simulink model "ProcessFlowRateModel_symbotic"  (Simulink 7.9)
settings: Solver=VariableStepDiscrete  StartTime=0.0  StopTime=100000  RelTol=1e-3
libraries: simeventslib x4
settings Model: Creator=tsprock3  LastModifiedBy=tsprock3
settings DebuggingCC: SimStateOlderReleaseMsg=warning

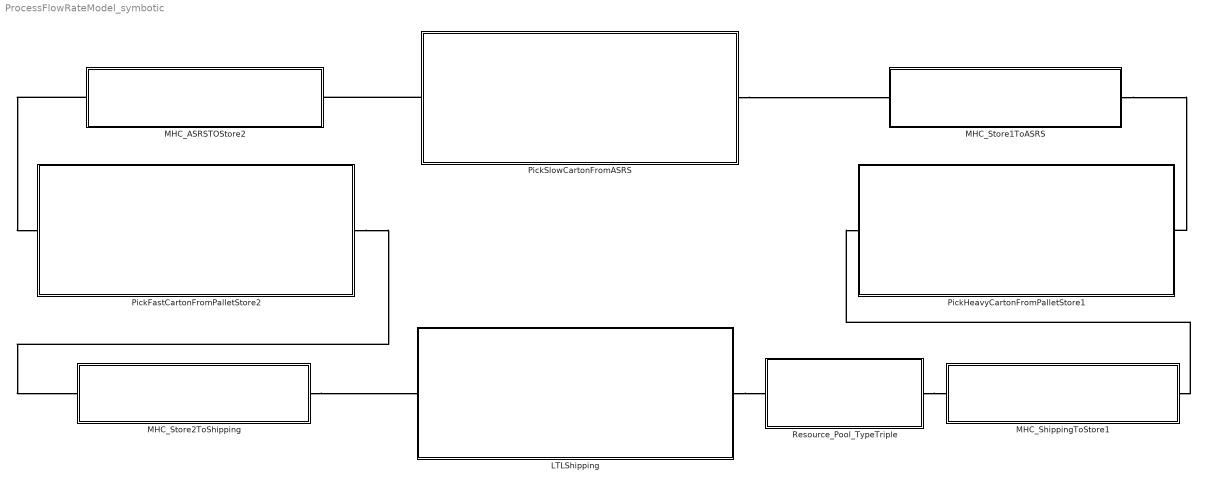
== system ProcessFlowRateModel_symbotic ==
  LTLShipping : Subsystem
  MHC_ASRSTOStore2 : Subsystem
  MHC_ShippingToStore1 : Subsystem
  MHC_Store1ToASRS : Subsystem
  MHC_Store2ToShipping : Subsystem
  PickFastCartonFromPalletStore2 : Subsystem
  PickHeavyCartonFromPalletStore1 : Subsystem
  PickSlowCartonFromASRS : Subsystem
  Resource_Pool_TypeTriple : Subsystem  mask{Quantity=25}
      mask prompts: Quantity "How many entities in resource pool?"
  connections:
  MHC_Store2ToShipping/RConn1 -- LTLShipping/LConn1
  MHC_ShippingToStore1/RConn1 -- PickHeavyCartonFromPalletStore1/LConn1
  MHC_Store1ToASRS/LConn1 -- PickHeavyCartonFromPalletStore1/RConn1
  PickFastCartonFromPalletStore2/RConn1 -- MHC_Store2ToShipping/LConn1
  MHC_ASRSTOStore2/RConn1 -- PickFastCartonFromPalletStore2/LConn1
  LTLShipping/RConn1 -- Resource_Pool_TypeTriple/RConn1
  Resource_Pool_TypeTriple/LConn1 -- MHC_ShippingToStore1/LConn1
  PickSlowCartonFromASRS/RConn1 -- MHC_ASRSTOStore2/LConn1
  PickSlowCartonFromASRS/LConn1 -- MHC_Store1ToASRS/RConn1

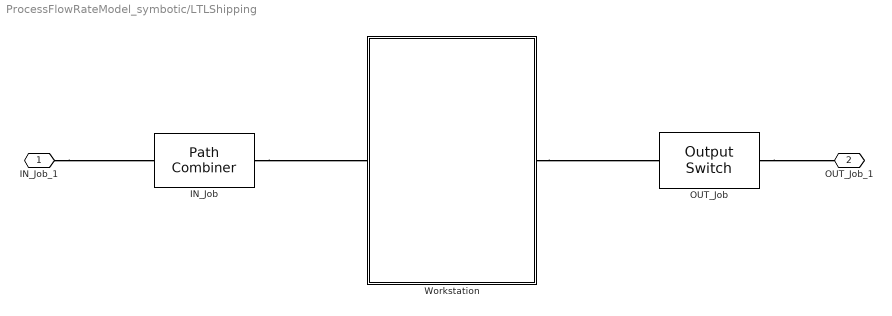
== system ProcessFlowRateModel_symbotic/LTLShipping ==
  IN_Job : PathCombiner  NumberInputPorts=1
  OUT_Job : OutputSwitch  NumberOutputPorts=1  SwitchingCriterion=Equiprobable  InitialSeed=15948
  Workstation : Subsystem
  IN_Job_1 : PMIOPort  Port=1  Side=Left
  OUT_Job_1 : PMIOPort  Port=2  Side=Right
  connections:
  IN_Job/RConn1 -- Workstation/LConn1
  Workstation/RConn1 -- OUT_Job/LConn1
  IN_Job_1/RConn1 -- IN_Job/LConn1
  OUT_Job/RConn1 -- OUT_Job_1/RConn1

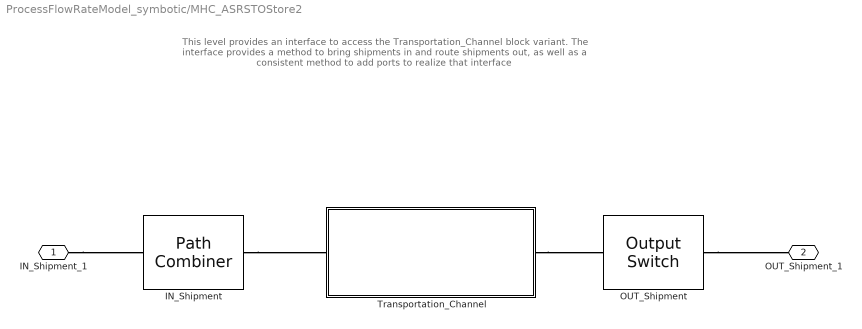
== system ProcessFlowRateModel_symbotic/MHC_ASRSTOStore2 ==
  note: This level provides an interface to access the Transportation_Channel block variant. The interface provides a method to
      | bring shipments in and route shipments out, as well as a consistent method to add ports to realize that interface
  IN_Shipment : PathCombiner  NumberInputPorts=1
  OUT_Shipment : OutputSwitch  NumberOutputPorts=1  AttributeName=Customer
  Transportation_Channel : Subsystem
  IN_Shipment_1 : PMIOPort  Port=1  Side=Left
  OUT_Shipment_1 : PMIOPort  Port=2  Side=Right
  connections:
  IN_Shipment/RConn1 -- Transportation_Channel/LConn1
  Transportation_Channel/RConn1 -- OUT_Shipment/LConn1
  IN_Shipment_1/RConn1 -- IN_Shipment/LConn1
  OUT_Shipment/RConn1 -- OUT_Shipment_1/RConn1

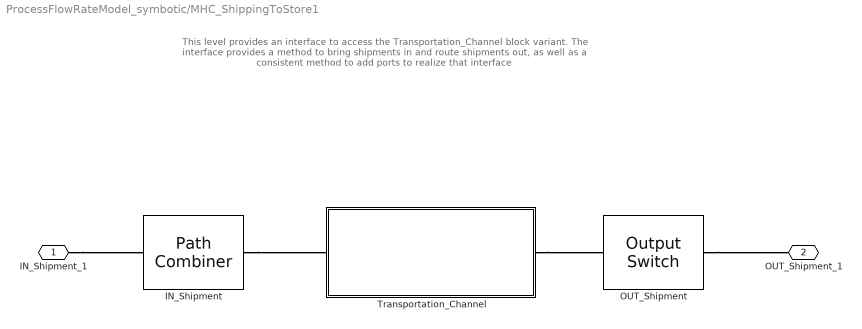
== system ProcessFlowRateModel_symbotic/MHC_ShippingToStore1 ==
  note: This level provides an interface to access the Transportation_Channel block variant. The interface provides a method to
      | bring shipments in and route shipments out, as well as a consistent method to add ports to realize that interface
  IN_Shipment : PathCombiner  NumberInputPorts=1
  OUT_Shipment : OutputSwitch  NumberOutputPorts=1  AttributeName=Customer
  Transportation_Channel : Subsystem
  IN_Shipment_1 : PMIOPort  Port=1  Side=Left
  OUT_Shipment_1 : PMIOPort  Port=2  Side=Right
  connections:
  IN_Shipment/RConn1 -- Transportation_Channel/LConn1
  Transportation_Channel/RConn1 -- OUT_Shipment/LConn1
  IN_Shipment_1/RConn1 -- IN_Shipment/LConn1
  OUT_Shipment/RConn1 -- OUT_Shipment_1/RConn1

== system ProcessFlowRateModel_symbotic/MHC_Store1ToASRS ==
  note: This level provides an interface to access the Transportation_Channel block variant. The interface provides a method to
      | bring shipments in and route shipments out, as well as a consistent method to add ports to realize that interface
  IN_Shipment : PathCombiner  NumberInputPorts=1
  OUT_Shipment : OutputSwitch  NumberOutputPorts=1  AttributeName=Customer
  Transportation_Channel : Subsystem
  IN_Shipment_1 : PMIOPort  Port=1  Side=Left
  OUT_Shipment_1 : PMIOPort  Port=2  Side=Right
  connections:
  IN_Shipment/RConn1 -- Transportation_Channel/LConn1
  Transportation_Channel/RConn1 -- OUT_Shipment/LConn1
  IN_Shipment_1/RConn1 -- IN_Shipment/LConn1
  OUT_Shipment/RConn1 -- OUT_Shipment_1/RConn1

== system ProcessFlowRateModel_symbotic/MHC_Store2ToShipping ==
  note: This level provides an interface to access the Transportation_Channel block variant. The interface provides a method to
      | bring shipments in and route shipments out, as well as a consistent method to add ports to realize that interface
  IN_Shipment : PathCombiner  NumberInputPorts=1
  OUT_Shipment : OutputSwitch  NumberOutputPorts=1  AttributeName=Customer
  Transportation_Channel : Subsystem
  IN_Shipment_1 : PMIOPort  Port=1  Side=Left
  OUT_Shipment_1 : PMIOPort  Port=2  Side=Right
  connections:
  IN_Shipment/RConn1 -- Transportation_Channel/LConn1
  Transportation_Channel/RConn1 -- OUT_Shipment/LConn1
  IN_Shipment_1/RConn1 -- IN_Shipment/LConn1
  OUT_Shipment/RConn1 -- OUT_Shipment_1/RConn1

== system ProcessFlowRateModel_symbotic/PickFastCartonFromPalletStore2 ==
  IN_Job : PathCombiner  NumberInputPorts=1
  OUT_Job : OutputSwitch  NumberOutputPorts=1  SwitchingCriterion=Equiprobable  InitialSeed=12731
  Workstation : Subsystem
  IN_Job_1 : PMIOPort  Port=1  Side=Left
  OUT_Job_1 : PMIOPort  Port=2  Side=Right
  connections:
  IN_Job/RConn1 -- Workstation/LConn1
  Workstation/RConn1 -- OUT_Job/LConn1
  IN_Job_1/RConn1 -- IN_Job/LConn1
  OUT_Job/RConn1 -- OUT_Job_1/RConn1

== system ProcessFlowRateModel_symbotic/PickHeavyCartonFromPalletStore1 ==
  IN_Job : PathCombiner  NumberInputPorts=1
  OUT_Job : OutputSwitch  NumberOutputPorts=1  SwitchingCriterion=Equiprobable  InitialSeed=9514
  Workstation : Subsystem
  IN_Job_1 : PMIOPort  Port=1  Side=Left
  OUT_Job_1 : PMIOPort  Port=2  Side=Right
  connections:
  IN_Job/RConn1 -- Workstation/LConn1
  Workstation/RConn1 -- OUT_Job/LConn1
  IN_Job_1/RConn1 -- IN_Job/LConn1
  OUT_Job/RConn1 -- OUT_Job_1/RConn1

== system ProcessFlowRateModel_symbotic/PickSlowCartonFromASRS ==
  IN_Job : PathCombiner  NumberInputPorts=1
  OUT_Job : OutputSwitch  NumberOutputPorts=1  SwitchingCriterion=Equiprobable  InitialSeed=9514
  Workstation : Subsystem
  IN_Job_1 : PMIOPort  Port=1  Side=Left
  OUT_Job_1 : PMIOPort  Port=2  Side=Right
  connections:
  IN_Job/RConn1 -- Workstation/LConn1
  Workstation/RConn1 -- OUT_Job/LConn1
  IN_Job_1/RConn1 -- IN_Job/LConn1
  OUT_Job/RConn1 -- OUT_Job_1/RConn1

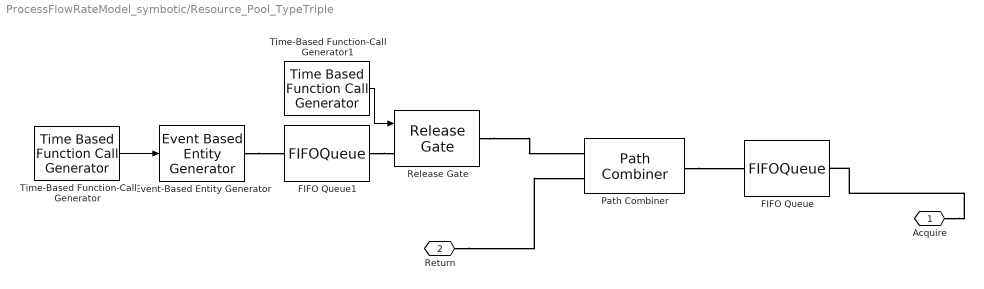
== system ProcessFlowRateModel_symbotic/Resource_Pool_TypeTriple ==
  Event-Based Entity Generator : EventBasedEntityGenerator  GenerateEntitiesUpon=Function call from port fcn
  FIFO Queue : FIFOQueue  Capacity=inf
  FIFO Queue1 : FIFOQueue  Capacity=inf
  Path Combiner : PathCombiner  NumberInputPorts=2
  Release Gate : ReleaseGate  OpenGateUpon=Function call from port fcn
  Time-Based Function-Call Generator : TimeBasedFunctionCallGenerator  EventGenerationMode=Only at simulation start  NumberOfEventsPerPeriod=Quantity
  Time-Based Function-Call Generator1 : TimeBasedFunctionCallGenerator
  Acquire : PMIOPort  Port=1  Side=Left
  Return : PMIOPort  Port=2  Side=Right
  wires:
  Time-Based Function-Call Generator/1 -> Event-Based Entity Generator/1
  Time-Based Function-Call Generator1/1 -> Release Gate/1
  connections:
  Path Combiner/RConn1 -- FIFO Queue/LConn1
  Return/RConn1 -- Path Combiner/LConn2
  Acquire/RConn1 -- FIFO Queue/RConn1
  Event-Based Entity Generator/RConn1 -- FIFO Queue1/LConn1
  Release Gate/RConn1 -- Path Combiner/LConn1
  FIFO Queue1/RConn1 -- Release Gate/LConn1

== system ProcessFlowRateModel_symbotic/LTLShipping/Workstation ==
  Shipping : Subsystem
  OUT_Job_1 : PMIOPort  Port=1  Side=Right
  IN_Job_1 : PMIOPort  Port=2  Side=Left
  connections:
  Shipping/RConn1 -- OUT_Job_1/RConn1
  IN_Job_1/RConn1 -- Shipping/LConn1

== system ProcessFlowRateModel_symbotic/MHC_ASRSTOStore2/Transportation_Channel ==
  FIFO Queue : FIFOQueue  Capacity=inf
  N-Server : NServer  NumberOfServers=inf  ServiceTime=10
  IN_Shipment : PMIOPort  Port=1  Side=Left
  OUT_Shipment : PMIOPort  Port=2  Side=Right
  connections:
  FIFO Queue/RConn1 -- N-Server/LConn1
  IN_Shipment/RConn1 -- FIFO Queue/LConn1
  OUT_Shipment/RConn1 -- N-Server/RConn1

== system ProcessFlowRateModel_symbotic/MHC_ShippingToStore1/Transportation_Channel ==
  FIFO Queue : FIFOQueue  Capacity=inf
  N-Server : NServer  NumberOfServers=inf  ServiceTime=20
  IN_Shipment : PMIOPort  Port=1  Side=Left
  OUT_Shipment : PMIOPort  Port=2  Side=Right
  connections:
  FIFO Queue/RConn1 -- N-Server/LConn1
  IN_Shipment/RConn1 -- FIFO Queue/LConn1
  OUT_Shipment/RConn1 -- N-Server/RConn1

== system ProcessFlowRateModel_symbotic/MHC_Store1ToASRS/Transportation_Channel ==
  FIFO Queue : FIFOQueue  Capacity=inf
  N-Server : NServer  NumberOfServers=inf  ServiceTime=10
  IN_Shipment : PMIOPort  Port=1  Side=Left
  OUT_Shipment : PMIOPort  Port=2  Side=Right
  connections:
  FIFO Queue/RConn1 -- N-Server/LConn1
  IN_Shipment/RConn1 -- FIFO Queue/LConn1
  OUT_Shipment/RConn1 -- N-Server/RConn1

== system ProcessFlowRateModel_symbotic/MHC_Store2ToShipping/Transportation_Channel ==
  FIFO Queue : FIFOQueue  Capacity=inf
  N-Server : NServer  NumberOfServers=inf  ServiceTime=20
  IN_Shipment : PMIOPort  Port=1  Side=Left
  OUT_Shipment : PMIOPort  Port=2  Side=Right
  connections:
  FIFO Queue/RConn1 -- N-Server/LConn1
  IN_Shipment/RConn1 -- FIFO Queue/LConn1
  OUT_Shipment/RConn1 -- N-Server/RConn1

== system ProcessFlowRateModel_symbotic/PickFastCartonFromPalletStore2/Workstation ==
  CartonPick : Subsystem
  OUT_Job_1 : PMIOPort  Port=1  Side=Right
  IN_Job_1 : PMIOPort  Port=2  Side=Left
  connections:
  IN_Job_1/RConn1 -- CartonPick/LConn1
  CartonPick/RConn1 -- OUT_Job_1/RConn1

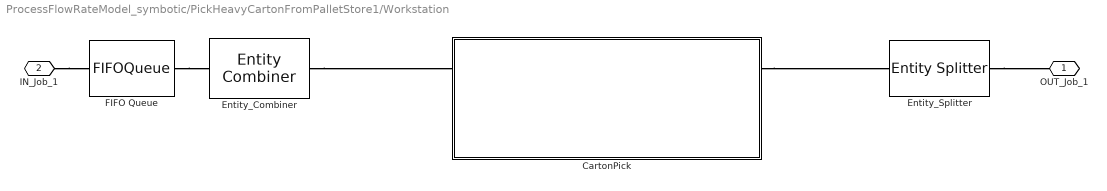
== system ProcessFlowRateModel_symbotic/PickHeavyCartonFromPalletStore1/Workstation ==
  CartonPick : Subsystem
  Entity_Combiner : EntityCombiner  NumberInputPorts=1
  Entity_Splitter : EntitySplitter  NumberOutputPorts=1
  FIFO Queue : FIFOQueue
  OUT_Job_1 : PMIOPort  Port=1  Side=Right
  IN_Job_1 : PMIOPort  Port=2  Side=Left
  connections:
  FIFO Queue/RConn1 -- Entity_Combiner/LConn1
  Entity_Splitter/RConn1 -- OUT_Job_1/RConn1
  IN_Job_1/RConn1 -- FIFO Queue/LConn1
  Entity_Combiner/RConn1 -- CartonPick/LConn1
  CartonPick/RConn1 -- Entity_Splitter/LConn1

== system ProcessFlowRateModel_symbotic/PickSlowCartonFromASRS/Workstation ==
  CartonPick : Subsystem
  Output Switch : OutputSwitch  NumberOutputPorts=1
  Path Combiner : PathCombiner  NumberInputPorts=1
  OUT_Job_1 : PMIOPort  Port=1  Side=Right
  IN_Job_1 : PMIOPort  Port=2  Side=Left
  connections:
  Output Switch/RConn1 -- OUT_Job_1/RConn1
  IN_Job_1/RConn1 -- Path Combiner/LConn1
  Path Combiner/RConn1 -- CartonPick/LConn1
  CartonPick/RConn1 -- Output Switch/LConn1

== system ProcessFlowRateModel_symbotic/LTLShipping/Workstation/Shipping ==
  IN_Job : PathCombiner  NumberInputPorts=1
  OUT_Job : OutputSwitch  NumberOutputPorts=1  SwitchingCriterion=Equiprobable  InitialSeed=65399
  Process : Subsystem
  IN_Job_1 : PMIOPort  Port=1  Side=Left
  OUT_Job_1 : PMIOPort  Port=2  Side=Right
  connections:
  IN_Job/RConn1 -- Process/LConn1
  Process/RConn1 -- OUT_Job/LConn1
  IN_Job_1/RConn1 -- IN_Job/LConn1
  OUT_Job_1/RConn1 -- OUT_Job/RConn1

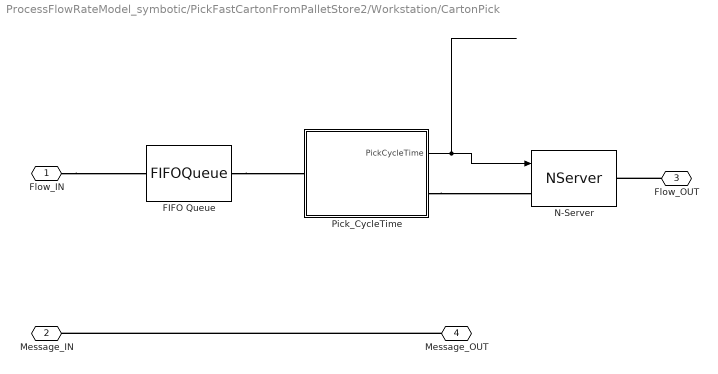
== system ProcessFlowRateModel_symbotic/PickFastCartonFromPalletStore2/Workstation/CartonPick ==
  FIFO Queue : FIFOQueue
  N-Server : NServer  NumberOfServers=inf  ServiceTimeFrom=Signal port t  ServiceTime=0
  Pick_CycleTime : Subsystem  mask{pickmean=5, pickstddev=0.25, traveltime=80, qty=20}
      mask prompts: pickmean "eachPickMean"; pickstddev "eachPickStdDev"; qty "carton_qty"
  Flow_IN : PMIOPort  Port=1  Side=Left
  Message_IN : PMIOPort  Port=2  Side=Left
  Flow_OUT : PMIOPort  Port=3  Side=Right
  Message_OUT : PMIOPort  Port=4  Side=Right
  wires:
  Pick_CycleTime/1(PickCycleTime) -> N-Server/1
  connections:
  Flow_IN/RConn1 -- FIFO Queue/LConn1
  Flow_OUT/RConn1 -- N-Server/RConn1
  Message_OUT/RConn1 -- Message_IN/RConn1
  FIFO Queue/RConn1 -- Pick_CycleTime/LConn1
  Pick_CycleTime/RConn1 -- N-Server/LConn1

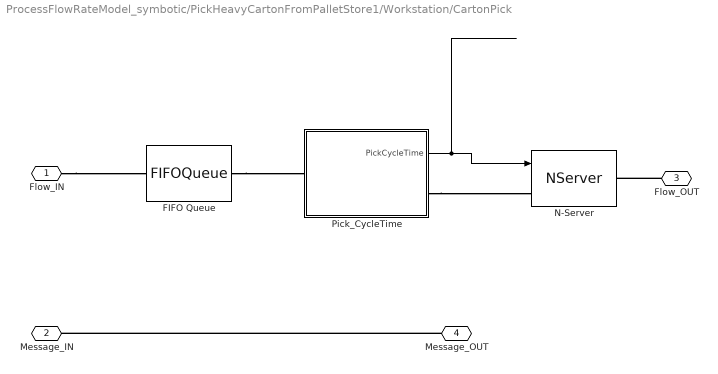
== system ProcessFlowRateModel_symbotic/PickHeavyCartonFromPalletStore1/Workstation/CartonPick ==
  FIFO Queue : FIFOQueue
  N-Server : NServer  NumberOfServers=inf  ServiceTimeFrom=Signal port t  ServiceTime=0
  Pick_CycleTime : Subsystem  mask{pickmean=5, pickstddev=0.25, traveltime=80, qty=20}
      mask prompts: pickmean "eachPickMean"; pickstddev "eachPickStdDev"; qty "carton_qty"
  Flow_IN : PMIOPort  Port=1  Side=Left
  Message_IN : PMIOPort  Port=2  Side=Left
  Flow_OUT : PMIOPort  Port=3  Side=Right
  Message_OUT : PMIOPort  Port=4  Side=Right
  wires:
  Pick_CycleTime/1(PickCycleTime) -> N-Server/1
  connections:
  Flow_IN/RConn1 -- FIFO Queue/LConn1
  Flow_OUT/RConn1 -- N-Server/RConn1
  Message_OUT/RConn1 -- Message_IN/RConn1
  FIFO Queue/RConn1 -- Pick_CycleTime/LConn1
  Pick_CycleTime/RConn1 -- N-Server/LConn1

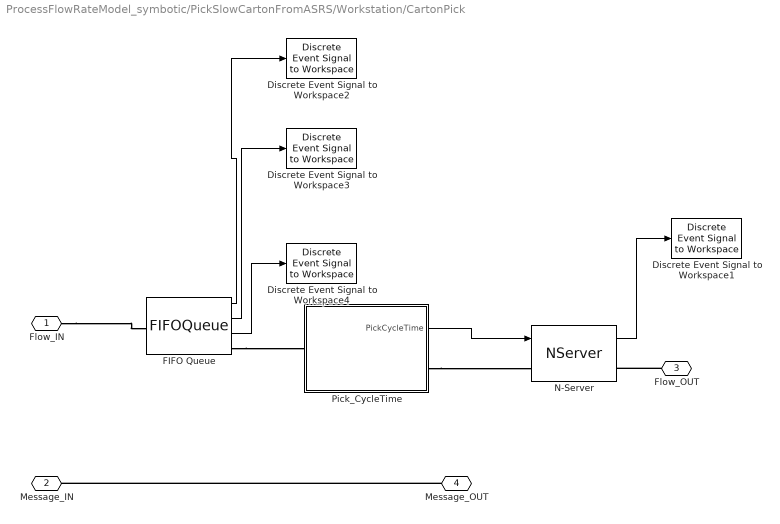
== system ProcessFlowRateModel_symbotic/PickSlowCartonFromASRS/Workstation/CartonPick ==
  Discrete Event Signal to Workspace1 : simeventslib/SimEvents Sinks/Discrete Event Signal to Workspace  VariableName=utilization  SaveFormat=Structure With Time  isMonitorOnly=off  isRecordIC=off
  Discrete Event Signal to Workspace2 : simeventslib/SimEvents Sinks/Discrete Event Signal to Workspace  VariableName=serviced_qty  SaveFormat=Structure With Time  isMonitorOnly=off  isRecordIC=off
  Discrete Event Signal to Workspace3 : simeventslib/SimEvents Sinks/Discrete Event Signal to Workspace  VariableName=num_wait  SaveFormat=Structure With Time  isMonitorOnly=off  isRecordIC=off
  Discrete Event Signal to Workspace4 : simeventslib/SimEvents Sinks/Discrete Event Signal to Workspace  VariableName=avg_wait  SaveFormat=Structure With Time  isMonitorOnly=off  isRecordIC=off
  FIFO Queue : FIFOQueue  StatNumberDeparted=on  StatNumberInBlock=on  StatAverageWait=on
      settings: OutputPortMap=o0,o1,o2
  N-Server : NServer  NumberOfServers=6  ServiceTimeFrom=Signal port t  ServiceTime=0  StatUtilization=on
      settings: OutputPortMap=o5
  Pick_CycleTime : Subsystem  mask{pickmean=5, pickstddev=0.25, traveltime=0, qty=60}
      mask prompts: pickmean "eachPickMean"; pickstddev "eachPickStdDev"; qty "carton_qty"
  Flow_IN : PMIOPort  Port=1  Side=Left
  Message_IN : PMIOPort  Port=2  Side=Left
  Flow_OUT : PMIOPort  Port=3  Side=Right
  Message_OUT : PMIOPort  Port=4  Side=Right
  wires:
  Pick_CycleTime/1(PickCycleTime) -> N-Server/1
  FIFO Queue/3 -> Discrete Event Signal to Workspace4/1
  FIFO Queue/2 -> Discrete Event Signal to Workspace3/1
  FIFO Queue/1 -> Discrete Event Signal to Workspace2/1
  N-Server/1 -> Discrete Event Signal to Workspace1/1
  connections:
  Flow_IN/RConn1 -- FIFO Queue/LConn1
  Flow_OUT/RConn1 -- N-Server/RConn1
  Message_OUT/RConn1 -- Message_IN/RConn1
  FIFO Queue/RConn1 -- Pick_CycleTime/LConn1
  Pick_CycleTime/RConn1 -- N-Server/LConn1

== system ProcessFlowRateModel_symbotic/LTLShipping/Workstation/Shipping/Process ==
  FIFO Queue : FIFOQueue  Capacity=inf
  N-Server : NServer  NumberOfServers=inf  ServiceTimeFrom=Signal port t
  ProcessTime : EventBasedRandomNumber  Distribution=Arbitrary discrete  minUnif=1  meanNorm=5  minUnid=29.9  maxUnid=30  numValueUnid=1  valueVecDisc=[0 30]  probVecDisc=[0 1]
  Job_OUT : PMIOPort  Port=1  Side=Right
  Job_IN : PMIOPort  Port=2  Side=Left
  wires:
  ProcessTime/1 -> N-Server/1
  connections:
  FIFO Queue/RConn1 -- N-Server/LConn1
  Job_OUT/RConn1 -- N-Server/RConn1
  Job_IN/RConn1 -- FIFO Queue/LConn1

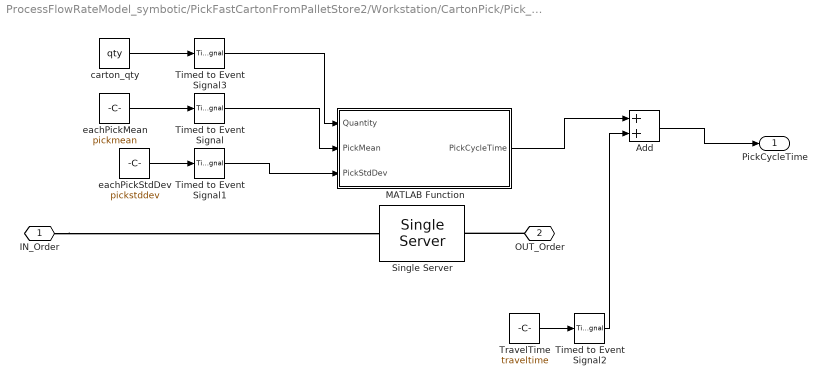
== system ProcessFlowRateModel_symbotic/PickFastCartonFromPalletStore2/Workstation/CartonPick/Pick_CycleTime ==
  Add : Sum
  MATLAB Function : MATLAB Function  TreatAsAtomicUnit=on
  Single Server : SingleServer  ServiceTime=0
  Timed to Event Signal{,1..3} (4 alike) : TimedToEventSignal
  TravelTime : Constant  Value=traveltime
  carton_qty : Constant  Value=qty
  eachPickMean : Constant  Value=pickmean
  eachPickStdDev : Constant  Value=pickstddev
  IN_Order : PMIOPort  Port=1  Side=Left
  OUT_Order : PMIOPort  Port=2  Side=Right
  PickCycleTime : Outport
  wires:
  MATLAB Function/1(PickCycleTime) -> Add/1
  Add/1 -> PickCycleTime/1
  eachPickStdDev/1 -> Timed to Event Signal1/1
  Timed to Event Signal1/1 -> MATLAB Function/3(PickStdDev)
  eachPickMean/1 -> Timed to Event Signal/1
  Timed to Event Signal/1 -> MATLAB Function/2(PickMean)
  TravelTime/1 -> Timed to Event Signal2/1
  Timed to Event Signal2/1 -> Add/2
  carton_qty/1 -> Timed to Event Signal3/1
  Timed to Event Signal3/1 -> MATLAB Function/1(Quantity)
  connections:
  OUT_Order/RConn1 -- Single Server/RConn1
  IN_Order/RConn1 -- Single Server/LConn1

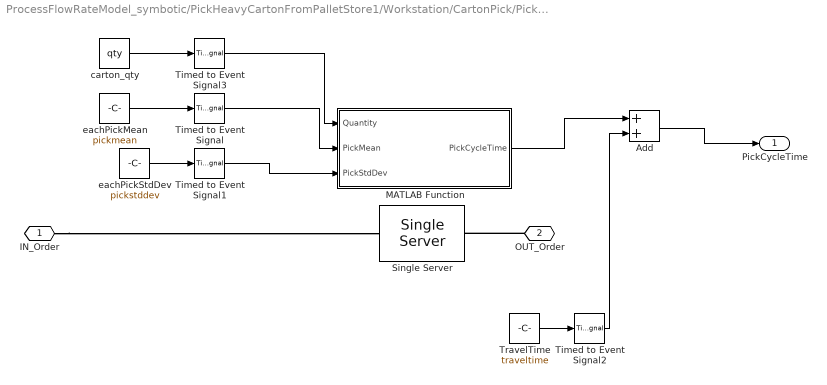
== system ProcessFlowRateModel_symbotic/PickHeavyCartonFromPalletStore1/Workstation/CartonPick/Pick_CycleTime ==
  Add : Sum
  MATLAB Function : MATLAB Function  TreatAsAtomicUnit=on
  Single Server : SingleServer  ServiceTime=0
  Timed to Event Signal{,1..3} (4 alike) : TimedToEventSignal
  TravelTime : Constant  Value=traveltime
  carton_qty : Constant  Value=qty
  eachPickMean : Constant  Value=pickmean
  eachPickStdDev : Constant  Value=pickstddev
  IN_Order : PMIOPort  Port=1  Side=Left
  OUT_Order : PMIOPort  Port=2  Side=Right
  PickCycleTime : Outport
  wires:
  MATLAB Function/1(PickCycleTime) -> Add/1
  Add/1 -> PickCycleTime/1
  eachPickStdDev/1 -> Timed to Event Signal1/1
  Timed to Event Signal1/1 -> MATLAB Function/3(PickStdDev)
  eachPickMean/1 -> Timed to Event Signal/1
  Timed to Event Signal/1 -> MATLAB Function/2(PickMean)
  TravelTime/1 -> Timed to Event Signal2/1
  Timed to Event Signal2/1 -> Add/2
  carton_qty/1 -> Timed to Event Signal3/1
  Timed to Event Signal3/1 -> MATLAB Function/1(Quantity)
  connections:
  OUT_Order/RConn1 -- Single Server/RConn1
  IN_Order/RConn1 -- Single Server/LConn1

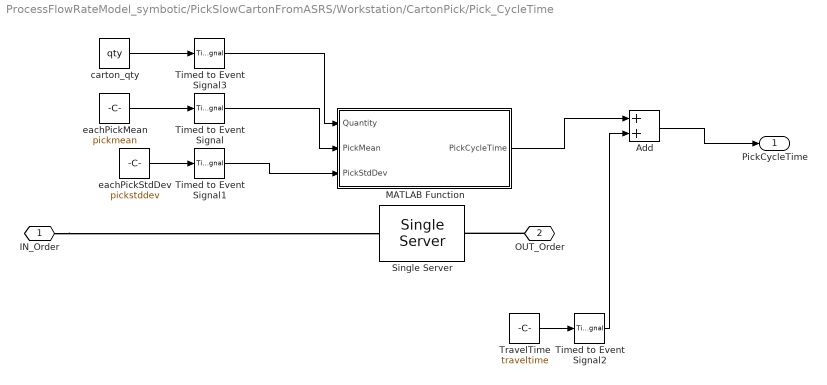
== system ProcessFlowRateModel_symbotic/PickSlowCartonFromASRS/Workstation/CartonPick/Pick_CycleTime ==
  Add : Sum
  MATLAB Function : MATLAB Function  TreatAsAtomicUnit=on
  Single Server : SingleServer  ServiceTime=0
  Timed to Event Signal{,1..3} (4 alike) : TimedToEventSignal
  TravelTime : Constant  Value=traveltime
  carton_qty : Constant  Value=qty
  eachPickMean : Constant  Value=pickmean
  eachPickStdDev : Constant  Value=pickstddev
  IN_Order : PMIOPort  Port=1  Side=Left
  OUT_Order : PMIOPort  Port=2  Side=Right
  PickCycleTime : Outport
  wires:
  MATLAB Function/1(PickCycleTime) -> Add/1
  Add/1 -> PickCycleTime/1
  eachPickStdDev/1 -> Timed to Event Signal1/1
  Timed to Event Signal1/1 -> MATLAB Function/3(PickStdDev)
  eachPickMean/1 -> Timed to Event Signal/1
  Timed to Event Signal/1 -> MATLAB Function/2(PickMean)
  TravelTime/1 -> Timed to Event Signal2/1
  Timed to Event Signal2/1 -> Add/2
  carton_qty/1 -> Timed to Event Signal3/1
  Timed to Event Signal3/1 -> MATLAB Function/1(Quantity)
  connections:
  OUT_Order/RConn1 -- Single Server/RConn1
  IN_Order/RConn1 -- Single Server/LConn1

== matlab function PickFastCartonFromPalletStore2/Workstation/CartonPick/Pick_CycleTime/MATLAB Function ==
  data: Quantity input double; PickCycleTime output double; PickMean input double; PickStdDev input double
function PickCycleTime = fcn(Quantity,  PickMean, PickStdDev)
%#codegen

coder.extrinsic('normrnd');
PickCycleTime = zeros(1, 'double');

Pick_Mean = Quantity*PickMean;
Pick_StdDev =Quantity*PickStdDev;

PickCycleTime = normrnd(Pick_Mean, sqrt(Pick_StdDev));

end

== matlab function PickHeavyCartonFromPalletStore1/Workstation/CartonPick/Pick_CycleTime/MATLAB Function ==
  data: Quantity input double; PickCycleTime output double; PickMean input double; PickStdDev input double
function PickCycleTime = fcn(Quantity,  PickMean, PickStdDev)
%#codegen

coder.extrinsic('normrnd');
PickCycleTime = zeros(1, 'double');

Pick_Mean = Quantity*PickMean;
Pick_StdDev =Quantity*PickStdDev;

PickCycleTime = normrnd(Pick_Mean, sqrt(Pick_StdDev));

end

== matlab function PickSlowCartonFromASRS/Workstation/CartonPick/Pick_CycleTime/MATLAB Function ==
  data: Quantity input double; PickCycleTime output double; PickMean input double; PickStdDev input double
function PickCycleTime = fcn(Quantity,  PickMean, PickStdDev)
%#codegen

coder.extrinsic('normrnd');
PickCycleTime = zeros(1, 'double');

Pick_Mean = Quantity*PickMean;
Pick_StdDev =Quantity*PickStdDev;

PickCycleTime = normrnd(Pick_Mean, sqrt(Pick_StdDev));

end
